simulink model "test_hand_simulink"  (R2022b)
settings: Solver=VariableStepAuto  StartTime=0.0  StopTime=10.0  RelTol=1e-3
InitFcn:
  | %Hand = hand;
values from neighbouring files (symbols this model uses):
  hand = create_hand_random('hand_IK_test', [2,2,2,4] )    [test_IK.m]    (also in test_hand.m = Hand('hand_exa'); test_hand_dynamics.m = create_hand_random('hand_with_VP_Mus', [2,2,2,4] ); test_hand_par_T.m = Hand('hand_exp'); test_obstacle_Set.m = create_hand_random('hand_Obstacle_Set', [1,2,0,0] ))
settings Model: Creator=ge26jow  LastModifiedBy=ge26jow

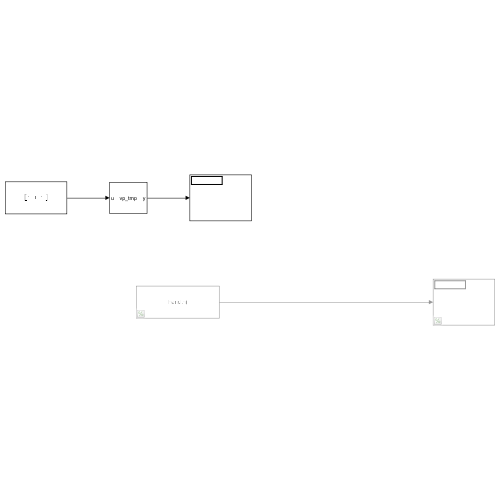
[thumbnail: Simulink's stored preview of the top-level diagram]
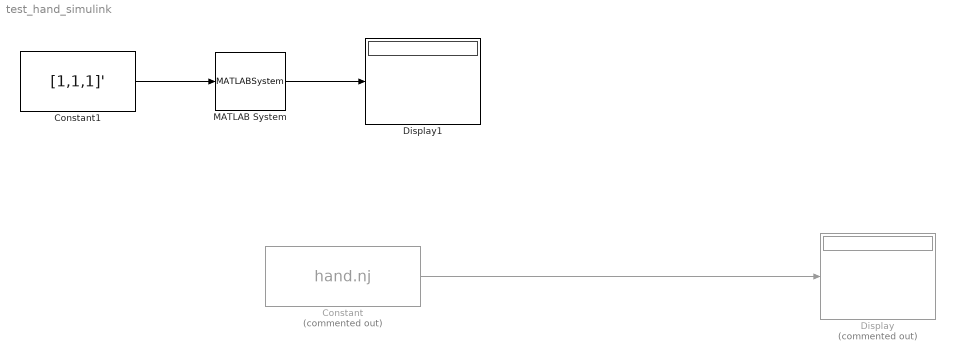
== system test_hand_simulink ==
  Constant : Constant  Commented=on  Value=hand.nj
  Constant1 : Constant  Value=[1,1,1]'
  Display : Display  Commented=on
  Display1 : Display
  MATLAB System : MATLABSystem  System=vp_tmp  link_p=[]  SimulateUsing=Code generation
      mask Type: vp_tmp
      mask Display:
      | disp('vp_tmp');
      | port_label('input',1,'u');
      | port_label('output',1,'y');
  wires:
  Constant/1 -> Display/1
  Constant1/1 -> MATLAB System/1
  MATLAB System/1 -> Display1/1
